simulink model "Resample_Block"  (Simulink 8.9)
settings: Solver=VariableStepAuto  StartTime=0.0  StopTime=0.001  RelTol=1e-3
settings Model: Creator=Alam  LastModifiedBy=Alam
settings DataIOCC: LimitDataPoints=off  SaveFormat=Dataset  SignalLoggingSaveFormat=Dataset
settings OptimizationCC: LifeSpan=auto
settings DebuggingCC: UnderspecifiedInitializationDetection=Simplified  MergeDetectMultiDrivingBlocksExec=error  FcnCallInpInsideContextMsg=error  StateNameClashWarn=none  SFUnexpectedBacktrackingDiag=error  SFNoUnconditionalDefaultTransitionDiag=error  SFExecutionAtInitializationDiag=warning
settings HardwareCC: ProdBitPerPointer=64  ProdBitPerSizeT=64  ProdBitPerPtrDiffT=64  ProdLargestAtomicFloat=Float  ProdIntDivRoundTo=Zero  ProdEndianess=LittleEndian  ProdWordSize=64  ProdHWDeviceType=Intel->x86-64 (Windows64)
settings ModelReferenceCC: PropagateSignalLabelsOutOfModel=on
settings GRTTargetCC: TargetLangStandard=C99 (ISO)  GeneratePreprocessorConditionals=Use local settings  CombineOutputUpdateFcns=on  GRTInterface=off
settings ConfigComp: CovMetricSettings=dwe  CovHtmlReporting=off  CovSaveCumulativeToWorkspaceVar=off  CovSaveSingleToWorkspaceVar=off  CovExternalEMLEnable=on

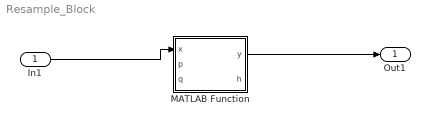
== system Resample_Block ==
  In1 : Inport  PortDimensions=[1 38192]
  MATLAB Function : MATLAB Function  TreatAsAtomicUnit=on  SystemSampleTime=0.002
  Out1 : Outport  PortDimensions=[1 32768]
  wires:
  In1/1 -> MATLAB Function/1(x)
  MATLAB Function/1(y) -> Out1/1

== matlab function MATLAB Function ==
  data: x input double; y output double; p input double; q input double; h output double
function  [y, h] = resampler( x, p, q)

bta = 5;  %--- design parameter for Kaiser window LPF
N = 10;

validateResampleRatio(p, q);

[p,q] = rat( p/q, 1e-12 );  %--- reduce to lowest terms 
   % (usually exact, sometimes not; loses at most 1 second every 10^12 seconds)
if (p==1) && (q==1)
    y = x; 
    h = 1;
    return
end
pqmax = max(p,q);
if length(N)>1      % use input filter
   L = length(N);
   h = N;
else                % design filter
   if( N>0 )
      fc = 1/2/pqmax;
      L = 2*N*pqmax + 1;
      h = firls( L-1, [0 2*fc 2*fc 1], [1 1 0 0]).*kaiser(L,bta)' ;
      h = p*h/sum(h);
   else
      L = p;
      h = ones(1,p);
   end
end

Lhalf = (L-1)/2;
isvect = any(size(x)==1);
if isvect
    Lx = length(x);
else
    Lx = size(x, 1);
end

% Need to delay output so that downsampling by q hits center tap of filter.
nz = floor(q-mod(Lhalf,q));
z = zeros(1,nz);
h = [z h(:).'];  % ensure that h is a row vector.
Lhalf = Lhalf + nz;

% Number of samples removed from beginning of output sequence 
% to compensate for delay of linear phase filter:
delay = floor(ceil(Lhalf)/q);

% Need to zero-pad so output length is exactly ceil(Lx*p/q).
nz1 = 0;
while ceil( ((Lx-1)*p+length(h)+nz1 )/q ) - delay < ceil(Lx*p/q)
    nz1 = nz1+1;
end
h = [h zeros(1,nz1)];
